simulink model "PTC_MBDS_CountDown_RE_Sample"  (R2013a)
settings: Solver=ode45  StartTime=0.0  StopTime=100  RelTol=1e-3
undefined symbols (not defined in the file): sigbuilder_block
libraries: simulink_extras x1, PTC_MBDS_LIB x1
settings Model: Creator=Jordan.Mosher  LastModifiedBy=sundeep.tuteja

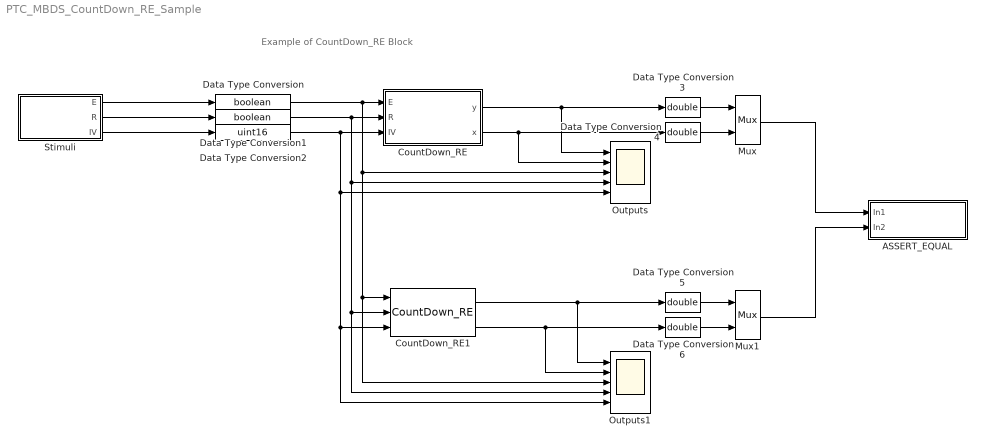
== system PTC_MBDS_CountDown_RE_Sample ==
  note: Example of CountDown_RE Block
  ASSERT_EQUAL : Subsystem
  CountDown_RE : Subsystem  InitFcn=|  mask(CountDown_RE){MBDS_LibraryBlock=on, E_Enabled=on, R_Enabled=on, IV_Enabled=on, IV=0, y_Enabled=on, x_Enabled=on, OutDataTypeStr=Inherit: Inherit via back propagation, MBDS_BlockVersion=05.40}
      | if(exist('MBDS_BlockCallback', 'file'))
      |    MBDS_BlockCallback('Update', gcb);
      | end
      mask prompts: MBDS_LibraryBlock "MBDS library block"; E_Enabled "Show E port"; R_Enabled "Show R port"; IV_Enabled "Show IV port"; IV "Initial value (IV):"; y_Enabled "Show y port"; x_Enabled "Show x port"; OutDataTypeStr "Output data type:"; MBDS_BlockVersion "Block version:"
      mask help: The output is true, if the number of block evaluations since the last reset is less than the initial number of block evaluations IV.
      mask init:
      | if(exist('MBDS_BlockCallback', 'file'))
      |    MBDS_BlockCallback('Init', gcb);
      | else
      |    % Disable all mask parameters
      |    MaskEnables = get_param(gcb, 'MaskEnables');
      |    for k = [1:length(MaskEnables)]
      |       MaskEnables{k} = 'off';
      |    end
      |    if(~isequal(MaskEnables, get_param(gcb, 'MaskEnables')))
      |       set_param(gcb, 'MaskEnables', MaskEnables);
      |    end
      | end
      mask Help: eval(['open([workdir(''library_dir:''),''\Blockset\help\'',get_param(gcb,''MaskType''),''.html''])'])
      mask Callback R_Enabled:
      | % Update mask parameter dialog
      | if(exist('MBDS_BlockCallback', 'file'))
      |    MBDS_BlockCallback('R_Enabled', gcb);
      | end
      mask Callback IV_Enabled:
      | % Update mask parameter dialog
      | if(exist('MBDS_BlockCallback', 'file'))
      |    MBDS_BlockCallback('IV_Enabled', gcb);
      | end
      mask Callback IV:
      | % Adopt Value
      | if(exist('MBDS_BlockCallback', 'file'))
      |    MBDS_BlockCallback('IV', gcb);
      | end
      mask Callback y_Enabled:
      | % Update mask parameter dialog
      | if(exist('MBDS_BlockCallback', 'file'))
      |    MBDS_BlockCallback('y_Enabled', gcb);
      | end
      mask Callback x_Enabled:
      | % Update mask parameter dialog
      | if(exist('MBDS_BlockCallback', 'file'))
      |    MBDS_BlockCallback('x_Enabled', gcb);
      | end
      mask TypeOptions OutDataTypeStr: Inherit: Inherit via back propagation | int8 | uint8 | int16 | uint16 | int32 | uint32
      mask Callback OutDataTypeStr:
      | % Configure data type
      | if(exist('MBDS_BlockCallback', 'file'))
      |    MBDS_BlockCallback('OutDataTypeStr', gcb);
      | end
      mask Display:
      | % Show icon or block text
      | if(exist('CountDown.tif', 'file'))
      |    image(imread('CountDown.tif','tif'), [0.295739348370927 0.17 0.378947368421053 0.66]);
      |    disp('')
      | else
      |    disp(sprintf('Count\nDown'));
      | end
      | 
      | % Display port labels
      | port_label('input', 1, 'E');
      | port_label('input', 2, 'R');
      | port_label('input', 3, 'IV');
      | port_label('output', 1, 'y');
      | port_label('output', 2, 'x');
  CountDown_RE1 : PTC_MBDS_LIB/MBDS Standard Library/Extended Operations/Counter & Timer/CountDown_RE  E_Enabled=on  R_Enabled=on  IV_Enabled=on  IV=0  y_Enabled=on  x_Enabled=on  OutDataTypeStr=Inherit: Inherit via back propagation  PTC_MBDS_BlockVersion=5.32  PTC_BlockType=PTC_MBDS_CountDown_RE
  Data Type Conversion : DataTypeConversion  InitFcn=|  OutDataTypeStr=boolean  SaturateOnIntegerOverflow=on
      | try
      |    MBDS_BlockCallback('Update', gcb);
      | end
  Data Type Conversion1 : DataTypeConversion  InitFcn=|  OutDataTypeStr=boolean  SaturateOnIntegerOverflow=on
      | try
      |    MBDS_BlockCallback('Update', gcb);
      | end
  Data Type Conversion2 : DataTypeConversion  InitFcn=|  OutDataTypeStr=uint16  SaturateOnIntegerOverflow=on
      | try
      |    MBDS_BlockCallback('Update', gcb);
      | end
  Data Type Conversion{3..6} (4 alike) : DataTypeConversion  OutDataTypeStr=double
  Mux : Mux  Inputs=2
  Mux1 : Mux  Inputs=2
  Outputs : Scope  NumInputPorts=5
      settings: TimeRange=100  YMin=0~0~0~15~-5  YMax=1~1~1~30~5  SampleInput=on  SampleTime=1
  Outputs1 : Scope  NumInputPorts=5
      settings: TimeRange=100  YMin=0~0~0~15~-5  YMax=1~1~1~30~5  SampleInput=on  SampleTime=1
  Stimuli : Subsystem  Tag=STV Subsys  LoadFcn=sigbuilder_block('load');  StartFcn=sigbuilder_block('start');  StopFcn=sigbuilder_block('stop');  ClipboardFcn=sigbuilder_block('clipboard');  mask(Sigbuilder block){}
      mask help: Sigbuilder GUI
      mask init:
      | if ~strcmp(get_param(bdroot(gcb),'SimulationStatus'),'stopped') tuvar = sigbuilder_block('maskInit'); end
      settings: CopyFcn=sigbuilder_block('copy');  DeleteFcn=sigbuilder_block('delete');  ModelCloseFcn=sigbuilder_block('modelClose');  PreSaveFcn=sigbuilder_block('preSave');  PauseFcn=sigbuilder_block('pause')  ContinueFcn=sigbuilder_block('continue')  NameChangeFcn=sigbuilder_block('namechange');  OpenFcn=sigbuilder_block('open',[66 294.75 404.25 223.5 ]);  CloseFcn=sigbuilder_block('close');
      mask Display: plot(0,0,100,100,[10,10,40,40,10],[80,20,20,80,80],[40,10],[50,50], [40,27,10],[65,72,56],[40,25,25,10],[28,28,43,43]);
  wires:
  Data Type Conversion/1 -> CountDown_RE/1(E), CountDown_RE1/1, Outputs1/3, Outputs/3
  Data Type Conversion1/1 -> CountDown_RE/2(R), CountDown_RE1/2, Outputs1/4, Outputs/4
  Data Type Conversion2/1 -> CountDown_RE/3(IV), CountDown_RE1/3, Outputs1/5, Outputs/5
  Stimuli/1(E) -> Data Type Conversion/1
  Stimuli/2(R) -> Data Type Conversion1/1
  Stimuli/3(IV) -> Data Type Conversion2/1
  CountDown_RE/1(y) -> Outputs/1, Data Type Conversion3/1
  CountDown_RE/2(x) -> Data Type Conversion4/1, Outputs/2
  CountDown_RE1/2 -> Outputs1/2, Data Type Conversion6/1
  CountDown_RE1/1 -> Data Type Conversion5/1, Outputs1/1
  Mux/1 -> ASSERT_EQUAL/1(In1)
  Mux1/1 -> ASSERT_EQUAL/2(In2)
  Data Type Conversion3/1 -> Mux/1
  Data Type Conversion4/1 -> Mux/2
  Data Type Conversion5/1 -> Mux1/1
  Data Type Conversion6/1 -> Mux1/2

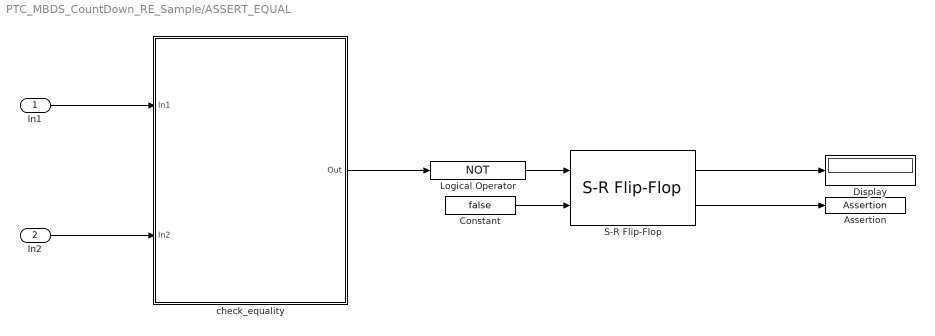
== system PTC_MBDS_CountDown_RE_Sample/ASSERT_EQUAL ==
  In1 : Inport
  In2 : Inport  Port=2
  Assertion : Assertion
  Constant : Constant  Value=false
  Display : Display
  Logical Operator : Logic  Operator=NOT  AllPortsSameDT=off  OutDataTypeStr=boolean
  S-R Flip-Flop : simulink_extras/Flip Flops/S-R Flip-Flop  initial_condition=0
  check_equality : MATLAB Function  TreatAsAtomicUnit=on
  wires:
  S-R Flip-Flop/1 -> Display/1
  check_equality/1(Out) -> Logical Operator/1
  Constant/1 -> S-R Flip-Flop/2
  S-R Flip-Flop/2 -> Assertion/1
  In2/1 -> check_equality/2(In2)
  In1/1 -> check_equality/1(In1)
  Logical Operator/1 -> S-R Flip-Flop/1

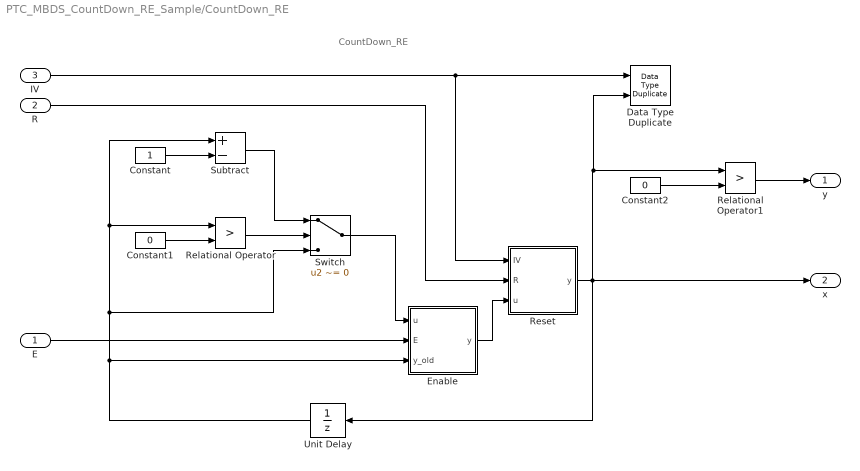
== system PTC_MBDS_CountDown_RE_Sample/CountDown_RE ==
  note: CountDown_RE
  E : Inport  OutDataTypeStr=boolean
  R : Inport  Port=2  OutDataTypeStr=boolean
  IV : Inport  Port=3
  Constant : Constant  OutDataTypeStr=Inherit: Inherit via back propagation
  Constant1 : Constant  Value=0  OutDataTypeStr=Inherit: Inherit via back propagation
  Constant2 : Constant  Value=0  OutDataTypeStr=Inherit: Inherit via back propagation
  Data Type Duplicate : DataTypeDuplicate
  Enable : Subsystem
  Relational Operator : RelationalOperator  Operator=>  OutDataTypeStr=boolean  InputSameDT=on
  Relational Operator1 : RelationalOperator  Operator=>  OutDataTypeStr=boolean  InputSameDT=on
  Reset : Subsystem
  Subtract : Sum  Inputs=+-  OutDataTypeStr=Inherit: Inherit via back propagation  SaturateOnIntegerOverflow=on  InputSameDT=on
  Switch : Switch  Criteria=u2 ~= 0  OutDataTypeStr=Inherit: Inherit via back propagation  InputSameDT=on
  Unit Delay : UnitDelay  SampleTime=-1
  y : Outport
  x : Outport  Port=2
  wires:
  E/1 -> Enable/2(E)
  R/1 -> Reset/2(R)
  IV/1 -> Reset/1(IV), Data Type Duplicate/1
  Reset/1(y) -> Relational Operator1/1, Data Type Duplicate/2, Unit Delay/1, x/1
  Constant2/1 -> Relational Operator1/2
  Relational Operator1/1 -> y/1
  Enable/1(y) -> Reset/3(u)
  Switch/1 -> Enable/1(u)
  Relational Operator/1 -> Switch/2
  Constant1/1 -> Relational Operator/2
  Subtract/1 -> Switch/1
  Constant/1 -> Subtract/2
  Unit Delay/1 -> Enable/3(y_old), Subtract/1, Relational Operator/1, Switch/3

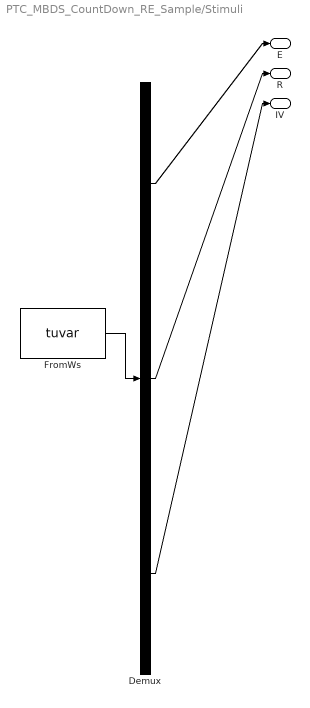
== system PTC_MBDS_CountDown_RE_Sample/Stimuli ==
  Demux : Demux  Tag=STV Demux  Outputs=3
  FromWs : FromWorkspace  Tag=STV FromWs  VariableName=tuvar  SampleTime=0  OutputAfterFinalValue=Holding final value
      SigBuilderData=|
      | common.afterFinalStr = 'Hold final value'
      | common.sampleTime = 0
      | dataSet.timeRange = [0 100]
      | dataSet.name = 'test data'
      | sbobj.Groups.Name = 'test data'
      | sbobj.Groups.Signals(1).Name = 'E'
      | sbobj.Groups.Signals(1).XData = [0 20 20 30 30 100]
      | sbobj.Groups.Signals(1).YData = [1 1 0 0 1 1]
      | sbobj.Groups.Signals(2).Name = 'R'
      | sbobj.Groups.Signals(2).XData = [0 9.5 9.5 10.5 10.5 60 60 70 70 100]
      | sbobj.Groups.Signals(2).YData = [0 0 1 1 0 0 1.02 1.02 0 0]
      | sbobj.Groups.Signals(3).Name = 'IV'
      | sbobj.Groups.Signals(3).XData = [0 60 60 100]
      | sbobj.Groups.Signals(3).YData = [19.95 19.95 30 30]
      | sbobj.Groups.TimeRange = [0 100]
  E : Outport  Tag=STV Outport
  R : Outport  Tag=STV Outport  Port=2
  IV : Outport  Tag=STV Outport  Port=3
  wires:
  Demux/3 -> IV/1
  Demux/2 -> R/1
  Demux/1 -> E/1
  FromWs/1 -> Demux/1

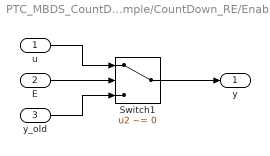
== system PTC_MBDS_CountDown_RE_Sample/CountDown_RE/Enable ==
  u : Inport
  E : Inport  Port=2
  y_old : Inport  Port=3
  Switch1 : Switch  Criteria=u2 ~= 0  OutDataTypeStr=Inherit: Inherit via back propagation  InputSameDT=on
  y : Outport
  wires:
  y_old/1 -> Switch1/3
  Switch1/1 -> y/1
  u/1 -> Switch1/1
  E/1 -> Switch1/2

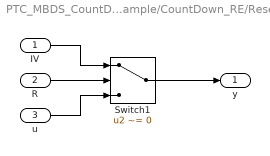
== system PTC_MBDS_CountDown_RE_Sample/CountDown_RE/Reset ==
  IV : Inport
  R : Inport  Port=2
  u : Inport  Port=3
  Switch1 : Switch  Criteria=u2 ~= 0  OutDataTypeStr=Inherit: Inherit via back propagation  InputSameDT=on
  y : Outport
  wires:
  u/1 -> Switch1/3
  Switch1/1 -> y/1
  IV/1 -> Switch1/1
  R/1 -> Switch1/2

== matlab function PTC_MBDS_CountDown_RE_Sample/ASSERT_EQUAL/check_equality ==
  data: In1 input; Out output; In2 input
function Out = check_equality(In1, In2)
%#codegen

Out = isequaln(In1, In2);

end
